simulink model "printer"  (R2017b)
settings: Solver=ode45  StartTime=0.0  StopTime=20  RelTol=1e-3  EnableMultiTasking=on
PreLoadFcn:
  | CONSTANTS
  | DEFAULT
  | System
  | Control
InitFcn:
  | CONSTANTS
  | DEFAULT
  | System
  | Control
values from neighbouring files (symbols this model uses):
  Amp0d = [C*L*R1 C*R1*R2]    [System.m]    (also in System_submitted.m = [Amp0d1 Amp0d0])
  Amp0n = [C*R1*R2-L]    [System.m]    (also in System_submitted.m = Amp0n0)
  Amp1d = Amp0d    [System.m]    (also in SystemHeadless.m; System_submitted.m)
  Amp1n = Amp0n    [System.m]    (also in SystemHeadless.m; System_submitted.m)
  AmpSat0 = MotorParam(NomV)    [System.m]    (also in SystemHeadless.m = q0(NomV); System_submitted.m = q0(NomV))
  AmpSat1 = Big    [System.m]    (also in SystemHeadless.m = AmpSat0; System_submitted.m = AmpSat0)
  BackEMF0 = 1/K_B    [System.m]    (also in SystemHeadless.m = 1 / q0(SpdK); System_submitted.m = 1 / q0(SpdK))
  BackEMF1 = 1/K_B1    [System.m]    (also in SystemHeadless.m = 1 / q1(SpdK); System_submitted.m = 1 / q1(SpdK))
  DegPerRad = 180/pi    (= 57.2957795131)    [CONSTANTS.m]
  Elec0d = [L_a R_a]    [System.m]    (also in SystemHeadless.m = [Elec0d1, Elec0d0]; System_submitted.m = [Elec0d1, Elec0d0])
  Elec0n = [1]    [System.m]    (also in SystemHeadless.m = 1; System_submitted.m = 1)
  Elec1d = [L_a R_a]    [System.m]    (also in SystemHeadless.m = [Elec1d1, Elec1d0]; System_submitted.m = [Elec1d1, Elec1d0])
  Elec1n = [1]    [System.m]    (also in SystemHeadless.m = 1; System_submitted.m = 1)
  JntSat1 = JntLim * RadPerDeg    [System.m]    (also in SystemHeadless.m = joint_limit; System_submitted.m = joint_limit)
  Mech0d = [J_system F_kf SpringK]    [System.m]    (also in SystemHeadless.m = [J_0, B_0, K_0]; System_submitted.m = [J_0, B_0, K_0])
  Mech0n = [1 0]    [System.m]    (also in SystemHeadless.m = [1, 0]; System_submitted.m = [1, 0])
  Mech1d = [J_rotor F_kf 0]    [System.m]    (also in SystemHeadless.m = [J_1, B_1, K_1]; System_submitted.m = [J_1, B_1, K_1])
  Mech1n = [1 0]    [System.m]    (also in SystemHeadless.m = [1, 0]; System_submitted.m = [1, 0])
  NomI0 = MotorParam(NomCurr)    [System.m]    (also in System_submitted.m = q0(NomCurr))
  NomI1 = MotorParam(NomCurr)    [System.m]    (also in System_submitted.m = q1(NomCurr))
  Sens0 = SensV / (SensAng * RadPerDeg)    [System.m]    (also in SystemHeadless.m; System_submitted.m)
  Sens1 = SensV / (SensAng * RadPerDeg)    [System.m]    (also in SystemHeadless.m; System_submitted.m)
  SensSat0 = SensV    [System.m]    (also in SystemHeadless.m; System_submitted.m)
  SensSat1 = SensV    [System.m]    (also in SystemHeadless.m; System_submitted.m)
  StallI0 = MotorParam(StallCurr)    [System.m]    (also in System_submitted.m = q0(StallCurr))
  StallI1 = MotorParam(StallCurr)    [System.m]    (also in System_submitted.m = q1(StallCurr))
  StFric0 = F_sf    [System.m]    (also in SystemHeadless.m = mu_SF * inner_fg; System_submitted.m = mu_SF * inner_fg)
  TConst0 = K_T    [System.m]    (also in SystemHeadless.m = q0(TorqueK); System_submitted.m = q0(TorqueK))
  TConst1 = K_T1    [System.m]    (also in SystemHeadless.m = q1(TorqueK); System_submitted.m = q1(TorqueK))
undefined symbols (not defined in the file or in its folder): FB0, FB1, Height, magnitude, PID0, PID1
libraries: simulink x22, vrlib x1
settings Model: Creator=Leos  LastModifiedBy=Moochster
settings DataIOCC: SaveFormat=Array
settings OptimizationCC: ExpressionDepthLimit=2147483647  LifeSpan=inf
settings DebuggingCC: UnderspecifiedInitializationDetection=Classic  MergeDetectMultiDrivingBlocksExec=none  SolverPrmCheckMsg=warning  FcnCallInpInsideContextMsg=warning  StateNameClashWarn=warning  SFUnexpectedBacktrackingDiag=warning  SFNoUnconditionalDefaultTransitionDiag=warning  SFExecutionAtInitializationDiag=none
settings HardwareCC: ProdBitPerPointer=32  ProdBitPerSizeT=32  ProdBitPerPtrDiffT=32  ProdLargestAtomicFloat=None  ProdIntDivRoundTo=Undefined  ProdEndianess=Unspecified  ProdWordSize=32  ProdHWDeviceType=32-bit Generic
settings ModelReferenceCC: PropagateSignalLabelsOutOfModel=off
settings CodeAppCC: StateflowObjectComments=on
settings GRTTargetCC: TargetLangStandard=C89/C90 (ANSI)  GeneratePreprocessorConditionals=Disable all  CombineOutputUpdateFcns=off  GRTInterface=on
settings ConfigComp: CovMetricSettings=dw  CovHtmlReporting=on  CovSaveCumulativeToWorkspaceVar=on  CovSaveSingleToWorkspaceVar=on  CovExternalEMLEnable=off  CovSFcnEnable=off

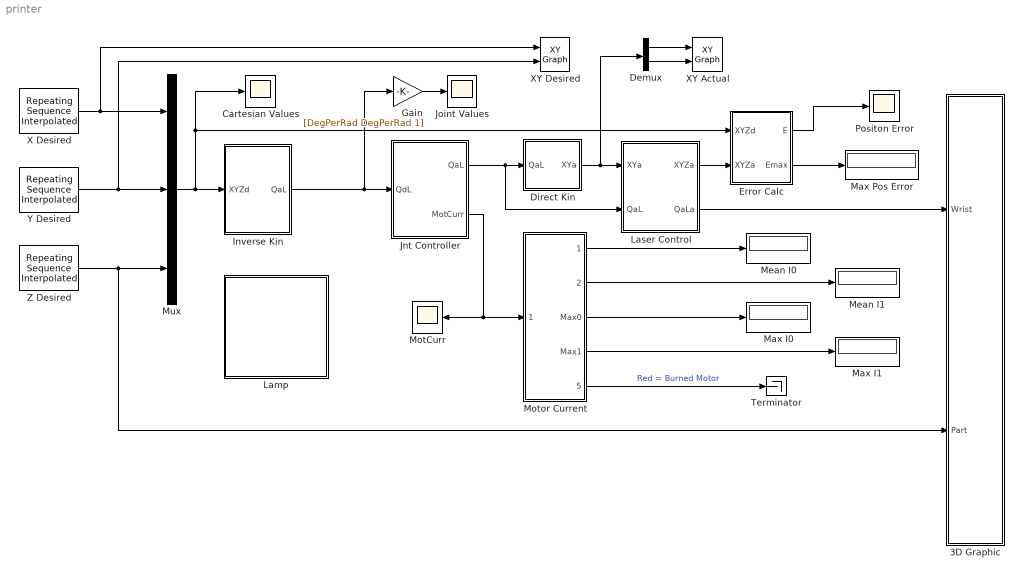
== system printer ==
  3D Graphic : Subsystem
  Cartesian Values : Scope
  Demux : Demux  Outputs=2
  Direct Kin : Subsystem
  Error Calc : Subsystem
  Gain : Gain  Gain=[DegPerRad DegPerRad 1]
  Inverse Kin : Subsystem
  Jnt Controller : Subsystem
  Joint Values : Scope
  Lamp : Subsystem  DialogController=hmiCreateDDGDialog  IsWebBlock=on  mask(MWDashboardBlock){webBlockId=7fcfd6b5-b98b-441a-9880-35fe4990fbef, webBlockType=lamp, ShowInLibBrowser=on, ShowInitialText=on, HMISrcModelName=printer}
      mask prompts: webBlockType "WebBlock Type"; HMISrcModelName "Source Model"
      mask help: SimulinkHMI:dialogs:LampDialogDesc
      mask Help: helpview([docroot '/mapfiles/simulink.map'], 'hmi_lamp')
      mask Display:
      | if strcmp(get_param(bdroot(gcb),'BlockDiagramType'), 'library')
      |     image([(matlabroot) '/toolbox/simulink/hmi/icons/Lamp.png']);
      | end
  Laser Control : Subsystem
  Max I0 : Display
  Max I1 : Display
  Max Pos Error : Display
  Mean I0 : Display
  Mean I1 : Display
  MotCurr : Scope
  Motor Current : Subsystem
  Mux : Mux  Inputs=3
  Positon Error : Scope
  Terminator : Terminator
  X Desired : simulink/Sources/Repeating Sequence Interpolated  OutValues=Xd  TimeValues=Time  LookUpMeth=Interpolation-Use End Values  tsamp=SampleTime  OutMin=[]  OutMax=[]  OutDataTypeStr=double  OutputDataTypeScalingMode=double  OutDataType=fixdt(0,8)  OutScaling=2^-10
  "XY Actual " : simulink/Sinks/XY Graph  xmin=-110  xmax=110  ymin=-110  ymax=110  st=-1
  XY Desired : simulink/Sinks/XY Graph  xmin=-110  xmax=110  ymin=-110  ymax=110  st=-1
  Y Desired : simulink/Sources/Repeating Sequence Interpolated  OutValues=Yd  TimeValues=Time  LookUpMeth=Interpolation-Use End Values  tsamp=SampleTime  OutMin=[]  OutMax=[]  OutDataTypeStr=double  OutputDataTypeScalingMode=double  OutDataType=fixdt(0,8)  OutScaling=2^-10
  Z Desired : simulink/Sources/Repeating Sequence Interpolated  OutValues=Zd  TimeValues=Time  LookUpMeth=Interpolation-Use End Values  tsamp=SampleTime  OutMin=[]  OutMax=[]  OutDataTypeStr=double  OutputDataTypeScalingMode=double  OutDataType=fixdt(0,8)  OutScaling=2^-10
  wires:
  Inverse Kin/1(QaL) -> Gain/1, Jnt Controller/1(QdL)
  Y Desired/1 -> XY Desired/2, Mux/2
  X Desired/1 -> Mux/1, XY Desired/1
  Demux/2 -> "XY Actual "/2
  Direct Kin/1(XYa) -> Demux/1, Laser Control/1(XYa)
  Demux/1 -> "XY Actual "/1
  Z Desired/1 -> 3D Graphic/2(Part), Mux/3
  Laser Control/2(QaLa) -> 3D Graphic/1(Wrist)
  Mux/1 -> Error Calc/1(XYZd), Cartesian Values/1, Inverse Kin/1(XYZd)
  Laser Control/1(XYZa) -> Error Calc/2(XYZa)
  Error Calc/2(Emax) -> Max Pos Error/1
  Error Calc/1(E) -> Positon Error/1
  Jnt Controller/2(MotCurr) -> MotCurr/1, Motor Current/1(MotCurr)
  Motor Current/1(Mean0) -> Mean I0/1
  Motor Current/4(Max1) -> Max I1/1
  Gain/1 -> Joint Values/1
  Motor Current/3(Max0) -> Max I0/1
  Motor Current/2(Mean1) -> Mean I1/1
  Motor Current/5(Burned) -> Terminator/1  "Red = Burned Motor"
  Jnt Controller/1(QaL) -> Direct Kin/1(QaL), Laser Control/2(QaL)

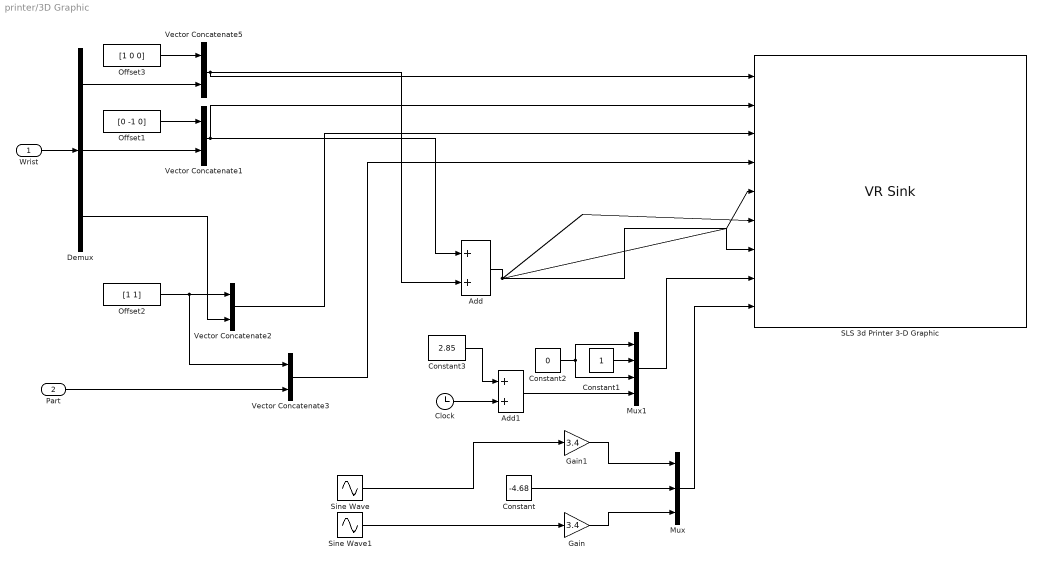
== system printer/3D Graphic ==
  Wrist : Inport
  Part : Inport  Port=2
  Add : Sum
  Add1 : Sum
  Clock : Clock
  Constant : Constant  Value=-4.68
  Constant1 : Constant
  Constant2 : Constant  Value=0
  Constant3 : Constant  Value=2.85
  Demux : Demux  Outputs=3
  Gain : Gain  Gain=3.4
  Gain1 : Gain  Gain=3.4
  Mux : Mux  Inputs=3
  Mux1 : Mux
  Offset1 : Constant  Value=[0 -1 0]
  Offset2 : Constant  Value=[1 1]
  Offset3 : Constant  Value=[1 0 0]
  SLS 3d Printer 3-D Graphic : vrlib/VR Sink  InstantiateOnLoad=on  SampleTime=0.01  ViewEnable=on  RemoteChange=off  RemoteView=off  FieldsWritten=q1.rotation.4.1.1.double#q2.rotation.4.1.1.double#LaserBeam.scale.3.1.1.double#Part.scale.3.1.1.double#HandL.rotation.4.1.1.double#ArmL.rotation.4.1.1.double#SleeveL.rotation.4.1.1.double#Fish.rotation.4.1.1.double#Fish.translation.3.1.1.double  WorldFileName=3dPrinter.WRL  AutoView=on  VideoDimensions=[]  AllowVariableSize=off
      settings: SourceProductBaseCode=VR
  Sine Wave : Sin  SampleTime=0
  Sine Wave1 : Sin  Phase=1.571  SampleTime=0
  Vector Concatenate{1..3,5} (4 alike) : Concatenate
  wires:
  Demux/1 -> Vector Concatenate5/2
  Demux/2 -> Vector Concatenate1/2
  Offset3/1 -> Vector Concatenate5/1
  Offset1/1 -> Vector Concatenate1/1
  Wrist/1 -> Demux/1
  Offset2/1 -> Vector Concatenate3/1, Vector Concatenate2/1
  Part/1 -> Vector Concatenate3/2
  Demux/3 -> Vector Concatenate2/2
  Vector Concatenate5/1 -> Add/2, SLS 3d Printer 3-D Graphic/1
  Vector Concatenate1/1 -> Add/1, SLS 3d Printer 3-D Graphic/2
  Vector Concatenate2/1 -> SLS 3d Printer 3-D Graphic/3
  Vector Concatenate3/1 -> SLS 3d Printer 3-D Graphic/4
  Add/1 -> SLS 3d Printer 3-D Graphic/5, SLS 3d Printer 3-D Graphic/6, SLS 3d Printer 3-D Graphic/7
  Constant/1 -> Mux/2
  Sine Wave/1 -> Gain1/1
  Sine Wave1/1 -> Gain/1
  Mux/1 -> SLS 3d Printer 3-D Graphic/9
  Constant1/1 -> Mux1/2
  Constant2/1 -> Mux1/3, Mux1/1
  Mux1/1 -> SLS 3d Printer 3-D Graphic/8
  Add1/1 -> Mux1/4
  Constant3/1 -> Add1/1
  Gain/1 -> Mux/3
  Gain1/1 -> Mux/1
  Clock/1 -> Add1/2

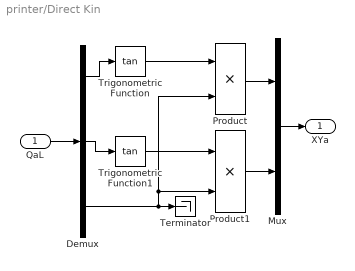
== system printer/Direct Kin ==
  QaL : Inport
  Demux : Demux  Outputs=3
  Mux : Mux  Inputs=2
  Product : Product
  Product1 : Product
  Terminator : Terminator
  Trigonometric Function : Trigonometry  Operator=tan
  Trigonometric Function1 : Trigonometry  Operator=tan
  XYa : Outport
  wires:
  QaL/1 -> Demux/1
  Mux/1 -> XYa/1
  Demux/1 -> Trigonometric Function/1
  Demux/2 -> Trigonometric Function1/1
  Demux/3 -> Terminator/1, Product/2, Product1/2
  Trigonometric Function/1 -> Product/1
  Product/1 -> Mux/1
  Product1/1 -> Mux/2
  Trigonometric Function1/1 -> Product1/1

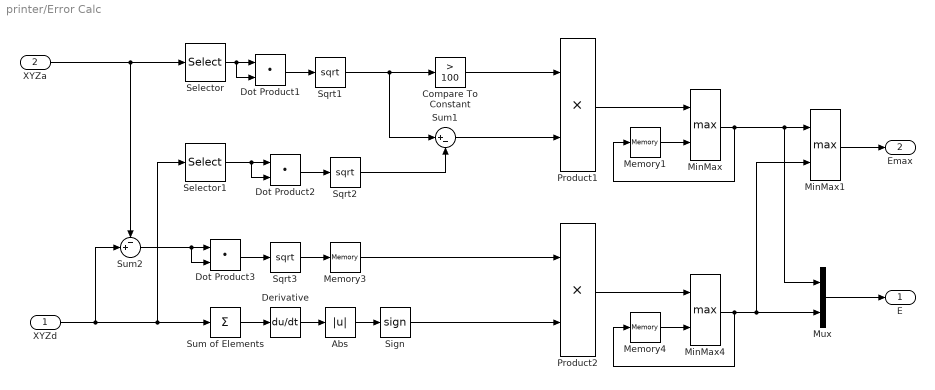
== system printer/Error Calc ==
  XYZd : Inport
  XYZa : Inport  Port=2
  Abs : Abs
  Compare To Constant : simulink/Logic and Bit Operations/Compare To Constant  relop=>  const=100  OutDataTypeStr=boolean
  Derivative : Derivative
  Dot Product1 : DotProduct  InputSameDT=on  OutDataTypeStr=Inherit: Inherit via internal rule
  Dot Product2 : DotProduct  InputSameDT=on  OutDataTypeStr=Inherit: Inherit via internal rule
  Dot Product3 : DotProduct  InputSameDT=on  OutDataTypeStr=Inherit: Inherit via internal rule
  Memory1 : Memory
  Memory3 : Memory
  Memory4 : Memory
  MinMax : MinMax  Function=max  Inputs=2
  MinMax1 : MinMax  Function=max  Inputs=2
  MinMax4 : MinMax  Function=max  Inputs=2
  Mux : Mux  Inputs=2
  Product1 : Product
  Product2 : Product
  Selector : Selector  InputPortWidth=3  IndexOptions=Index vector (dialog)  Indices=[1 2]  OutputSizes=1
  Selector1 : Selector  InputPortWidth=3  IndexOptions=Index vector (dialog)  Indices=[1 2]  OutputSizes=1
  Sign : Signum
  Sqrt1 : Sqrt  SaturateOnIntegerOverflow=on
  Sqrt2 : Sqrt  SaturateOnIntegerOverflow=on
  Sqrt3 : Sqrt  SaturateOnIntegerOverflow=on
  Sum of Elements : Sum  Inputs=+
  Sum1 : Sum  Inputs=|+-
  Sum2 : Sum  Inputs=-+|
  E : Outport
  Emax : Outport  Port=2
  wires:
  XYZd/1 -> Sum2/2, Selector1/1, Sum of Elements/1
  Derivative/1 -> Abs/1
  Abs/1 -> Sign/1
  Sum of Elements/1 -> Derivative/1
  Selector/1 -> Dot Product1/2, Dot Product1/1
  Dot Product1/1 -> Sqrt1/1
  XYZa/1 -> Sum2/1, Selector/1
  Sign/1 -> Product2/2
  Sqrt1/1 -> Sum1/1, Compare To Constant/1
  Product1/1 -> MinMax/1
  Compare To Constant/1 -> Product1/1
  Sum1/1 -> Product1/2
  Memory1/1 -> MinMax/2
  MinMax/1 -> Mux/1, MinMax1/1, Memory1/1
  Memory4/1 -> MinMax4/2
  Product2/1 -> MinMax4/1
  MinMax4/1 -> MinMax1/2, Mux/2, Memory4/1
  MinMax1/1 -> Emax/1
  Mux/1 -> E/1
  Memory3/1 -> Product2/1
  Selector1/1 -> Dot Product2/2, Dot Product2/1
  Dot Product2/1 -> Sqrt2/1
  Sqrt2/1 -> Sum1/2
  Sum2/1 -> Dot Product3/2, Dot Product3/1
  Dot Product3/1 -> Sqrt3/1
  Sqrt3/1 -> Memory3/1

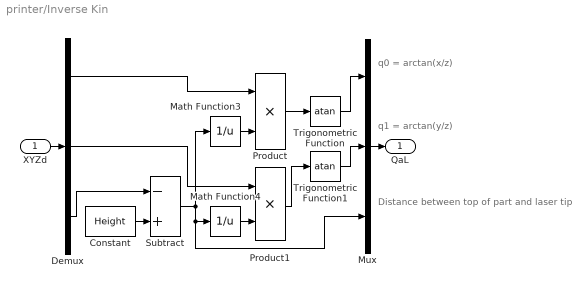
== system printer/Inverse Kin ==
  note: Distance between top of part and laser tip
  note: q0 = arctan(x/z)
  note: q1 = arctan(y/z)
  XYZd : Inport
  Constant : Constant  Value=Height
  Demux : Demux  Outputs=3
  Math Function3 : Math  Operator=reciprocal  SaturateOnIntegerOverflow=on
  Math Function4 : Math  Operator=reciprocal  SaturateOnIntegerOverflow=on
  Mux : Mux  Inputs=3
  Product : Product
  Product1 : Product
  Subtract : Sum  Inputs=-+
  Trigonometric Function : Trigonometry  Operator=atan
  Trigonometric Function1 : Trigonometry  Operator=atan
  QaL : Outport
  wires:
  XYZd/1 -> Demux/1
  Mux/1 -> QaL/1
  Demux/1 -> Product/1
  Demux/2 -> Product1/1
  Demux/3 -> Subtract/1
  Trigonometric Function/1 -> Mux/1
  Trigonometric Function1/1 -> Mux/2
  Constant/1 -> Subtract/2
  Product/1 -> Trigonometric Function/1
  Product1/1 -> Trigonometric Function1/1
  Math Function3/1 -> Product/2
  Math Function4/1 -> Product1/2
  Subtract/1 -> Math Function3/1, Math Function4/1, Mux/3

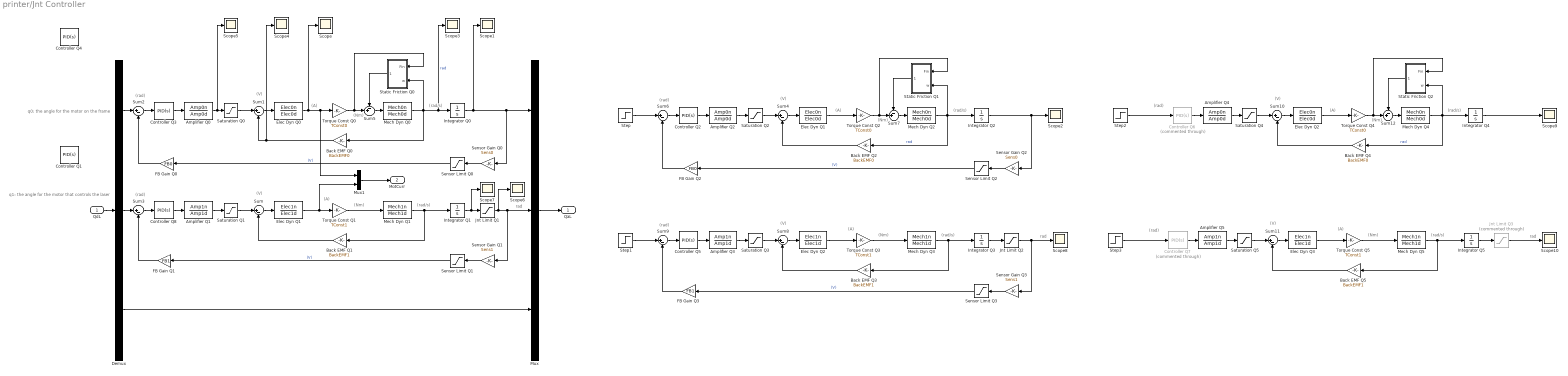
== system printer/Jnt Controller ==
  note: rad
  note: (rad/s)
  note: (V)
  note: (rad)
  note: (A)
  note: (Nm)
  note: (rad/s)
  note: (V)
  note: (rad)
  note: (A)
  note: (Nm)
  note: q0: the angle for the motor on the frame
  note: q1: the angle for the motor that controls the laser
  note: (Nm)
  note: (rad/s)
  note: (V)
  note: (rad)
  note: (A)
  note: (A)
  note: (rad)
  note: (V)
  note: (rad/s)
  note: rad
  note: (Nm)
  note: (A)
  note: (Nm)
  note: (rad)
  note: (rad/s)
  note: (V)
  note: (rad)
  note: (Nm)
  note: (A)
  note: rad
  note: (rad/s)
  note: (V)
  QdL : Inport
  Amplifier Q0 : TransferFcn  Numerator=Amp0n  Denominator=Amp0d
  Amplifier Q1 : TransferFcn  Numerator=Amp1n  Denominator=Amp1d
  Amplifier Q2 : TransferFcn  Numerator=Amp0n  Denominator=Amp0d
  Amplifier Q3 : TransferFcn  Numerator=Amp1n  Denominator=Amp1d
  Amplifier Q4 : TransferFcn  Numerator=Amp0n  Denominator=Amp0d
  Amplifier Q5 : TransferFcn  Numerator=Amp1n  Denominator=Amp1d
  Back EMF Q0 : Gain  Gain=BackEMF0
  Back EMF Q1 : Gain  Gain=BackEMF1
  Back EMF Q2 : Gain  Gain=BackEMF0
  Back EMF Q3 : Gain  Gain=BackEMF1
  Back EMF Q4 : Gain  Gain=BackEMF0
  Back EMF Q5 : Gain  Gain=BackEMF1
  Controller Q1 : simulink/Continuous/PID Controller  Controller=PID  TimeDomain=Continuous-time  SampleTime=-1  IntegratorMethod=Forward Euler  FilterMethod=Forward Euler  Form=Parallel  UseFilter=on  ControllerParametersSource=internal  P=0.325398300430713  I=1.13628459398882  D=0.0191166653473395  N=7531.30108660087  InitialConditionSource=internal  InitialConditionForIntegrator=0  InitialConditionForFilter=0  ExternalReset=none  LimitOutput=off  UpperSaturationLimit=inf  LowerSaturationLimit=-inf  LinearizeAsGain=on  AntiWindupMode=none  Kb=1  TrackingMode=off  Kt=1  PParamMin=[]  PParamMax=[]  IParamMin=[]  IParamMax=[]  DParamMin=[]  DParamMax=[]  NParamMin=[]  NParamMax=[]  KbParamMin=[]  KbParamMax=[]  KtParamMin=[]  KtParamMax=[]  POutMin=[]  POutMax=[]  IOutMin=[]  IOutMax=[]  DOutMin=[]  DOutMax=[]  NOutMin=[]  NOutMax=[]  KbOutMin=[]  KbOutMax=[]  KtOutMin=[]  KtOutMax=[]  IntegratorOutMin=[]  IntegratorOutMax=[]  FilterOutMin=[]  FilterOutMax=[]  SumOutMin=[]  SumOutMax=[]  SumI1OutMin=[]  SumI1OutMax=[]  SumI2OutMin=[]  SumI2OutMax=[]  SumI3OutMin=[]  SumI3OutMax=[]  SumDOutMin=[]  SumDOutMax=[]  SaturationOutMin=[]  SaturationOutMax=[]  IntegratorContinuousStateAttributes=''  IntegratorStateMustResolveToSignalObject=off  IntegratorRTWStateStorageClass=Auto  FilterContinuousStateAttributes=''  FilterStateMustResolveToSignalObject=off  FilterRTWStateStorageClass=Auto  DifferentiatorICPrevScaledInput=0  DifferentiatorOutMin=[]  DifferentiatorOutMax=[]  InitialConditionSetting=State (most efficient)  FilterDiffOutCoefMin=[]  FilterDiffOutCoefMax=[]  SumDenOutMin=[]  SumDenOutMax=[]  SumNumOutMin=[]  SumNumOutMax=[]  ReciprocalOutMin=[]  ReciprocalOutMax=[]  DivideOutMin=[]  DivideOutMax=[]  TunerSelectOption=Transfer Function Based (PID Tuner App)
  Controller Q2 : simulink/Continuous/PID Controller  Controller=PID  TimeDomain=Continuous-time  SampleTime=-1  IntegratorMethod=Forward Euler  FilterMethod=Forward Euler  Form=Parallel  UseFilter=on  ControllerParametersSource=internal  P=PID0(1)  I=PID0(2)  D=PID0(3)  N=100  InitialConditionSource=internal  InitialConditionForIntegrator=0  InitialConditionForFilter=0  ExternalReset=none  LimitOutput=off  UpperSaturationLimit=inf  LowerSaturationLimit=-inf  LinearizeAsGain=on  AntiWindupMode=none  Kb=1  TrackingMode=off  Kt=1  PParamMin=[]  PParamMax=[]  IParamMin=[]  IParamMax=[]  DParamMin=[]  DParamMax=[]  NParamMin=[]  NParamMax=[]  KbParamMin=[]  KbParamMax=[]  KtParamMin=[]  KtParamMax=[]  POutMin=[]  POutMax=[]  IOutMin=[]  IOutMax=[]  DOutMin=[]  DOutMax=[]  NOutMin=[]  NOutMax=[]  KbOutMin=[]  KbOutMax=[]  KtOutMin=[]  KtOutMax=[]  IntegratorOutMin=[]  IntegratorOutMax=[]  FilterOutMin=[]  FilterOutMax=[]  SumOutMin=[]  SumOutMax=[]  SumI1OutMin=[]  SumI1OutMax=[]  SumI2OutMin=[]  SumI2OutMax=[]  SumI3OutMin=[]  SumI3OutMax=[]  SumDOutMin=[]  SumDOutMax=[]  SaturationOutMin=[]  SaturationOutMax=[]  IntegratorContinuousStateAttributes=''  IntegratorStateMustResolveToSignalObject=off  IntegratorRTWStateStorageClass=Auto  FilterContinuousStateAttributes=''  FilterStateMustResolveToSignalObject=off  FilterRTWStateStorageClass=Auto  DifferentiatorICPrevScaledInput=0  DifferentiatorOutMin=[]  DifferentiatorOutMax=[]  InitialConditionSetting=State (most efficient)  FilterDiffOutCoefMin=[]  FilterDiffOutCoefMax=[]  SumDenOutMin=[]  SumDenOutMax=[]  SumNumOutMin=[]  SumNumOutMax=[]  ReciprocalOutMin=[]  ReciprocalOutMax=[]  DivideOutMin=[]  DivideOutMax=[]  TunerSelectOption=Transfer Function Based (PID Tuner App)
  Controller Q3 : simulink/Continuous/PID Controller  Controller=PID  TimeDomain=Continuous-time  SampleTime=-1  IntegratorMethod=Forward Euler  FilterMethod=Forward Euler  Form=Parallel  UseFilter=on  ControllerParametersSource=internal  P=PID0(1)  I=PID0(2)  D=PID0(3)  N=100  InitialConditionSource=internal  InitialConditionForIntegrator=0  InitialConditionForFilter=0  ExternalReset=none  LimitOutput=off  UpperSaturationLimit=inf  LowerSaturationLimit=-inf  LinearizeAsGain=on  AntiWindupMode=none  Kb=1  TrackingMode=off  Kt=1  PParamMin=[]  PParamMax=[]  IParamMin=[]  IParamMax=[]  DParamMin=[]  DParamMax=[]  NParamMin=[]  NParamMax=[]  KbParamMin=[]  KbParamMax=[]  KtParamMin=[]  KtParamMax=[]  POutMin=[]  POutMax=[]  IOutMin=[]  IOutMax=[]  DOutMin=[]  DOutMax=[]  NOutMin=[]  NOutMax=[]  KbOutMin=[]  KbOutMax=[]  KtOutMin=[]  KtOutMax=[]  IntegratorOutMin=[]  IntegratorOutMax=[]  FilterOutMin=[]  FilterOutMax=[]  SumOutMin=[]  SumOutMax=[]  SumI1OutMin=[]  SumI1OutMax=[]  SumI2OutMin=[]  SumI2OutMax=[]  SumI3OutMin=[]  SumI3OutMax=[]  SumDOutMin=[]  SumDOutMax=[]  SaturationOutMin=[]  SaturationOutMax=[]  IntegratorContinuousStateAttributes=''  IntegratorStateMustResolveToSignalObject=off  IntegratorRTWStateStorageClass=Auto  FilterContinuousStateAttributes=''  FilterStateMustResolveToSignalObject=off  FilterRTWStateStorageClass=Auto  DifferentiatorICPrevScaledInput=0  DifferentiatorOutMin=[]  DifferentiatorOutMax=[]  InitialConditionSetting=State (most efficient)  FilterDiffOutCoefMin=[]  FilterDiffOutCoefMax=[]  SumDenOutMin=[]  SumDenOutMax=[]  SumNumOutMin=[]  SumNumOutMax=[]  ReciprocalOutMin=[]  ReciprocalOutMax=[]  DivideOutMin=[]  DivideOutMax=[]  TunerSelectOption=Transfer Function Based (PID Tuner App)
  Controller Q4 : simulink/Continuous/PID Controller  Controller=PID  TimeDomain=Continuous-time  SampleTime=-1  IntegratorMethod=Forward Euler  FilterMethod=Forward Euler  Form=Parallel  UseFilter=on  ControllerParametersSource=internal  P=3.19495744260721  I=12.8018971006006  D=0.15685788274795  N=317.014850980507  InitialConditionSource=internal  InitialConditionForIntegrator=0  InitialConditionForFilter=0  ExternalReset=none  LimitOutput=off  UpperSaturationLimit=inf  LowerSaturationLimit=-inf  LinearizeAsGain=on  AntiWindupMode=none  Kb=1  TrackingMode=off  Kt=1  PParamMin=[]  PParamMax=[]  IParamMin=[]  IParamMax=[]  DParamMin=[]  DParamMax=[]  NParamMin=[]  NParamMax=[]  KbParamMin=[]  KbParamMax=[]  KtParamMin=[]  KtParamMax=[]  POutMin=[]  POutMax=[]  IOutMin=[]  IOutMax=[]  DOutMin=[]  DOutMax=[]  NOutMin=[]  NOutMax=[]  KbOutMin=[]  KbOutMax=[]  KtOutMin=[]  KtOutMax=[]  IntegratorOutMin=[]  IntegratorOutMax=[]  FilterOutMin=[]  FilterOutMax=[]  SumOutMin=[]  SumOutMax=[]  SumI1OutMin=[]  SumI1OutMax=[]  SumI2OutMin=[]  SumI2OutMax=[]  SumI3OutMin=[]  SumI3OutMax=[]  SumDOutMin=[]  SumDOutMax=[]  SaturationOutMin=[]  SaturationOutMax=[]  IntegratorContinuousStateAttributes=''  IntegratorStateMustResolveToSignalObject=off  IntegratorRTWStateStorageClass=Auto  FilterContinuousStateAttributes=''  FilterStateMustResolveToSignalObject=off  FilterRTWStateStorageClass=Auto  DifferentiatorICPrevScaledInput=0  DifferentiatorOutMin=[]  DifferentiatorOutMax=[]  InitialConditionSetting=State (most efficient)  FilterDiffOutCoefMin=[]  FilterDiffOutCoefMax=[]  SumDenOutMin=[]  SumDenOutMax=[]  SumNumOutMin=[]  SumNumOutMax=[]  ReciprocalOutMin=[]  ReciprocalOutMax=[]  DivideOutMin=[]  DivideOutMax=[]  TunerSelectOption=Transfer Function Based (PID Tuner App)
  Controller Q5 : simulink/Continuous/PID Controller  Controller=PID  TimeDomain=Continuous-time  SampleTime=-1  IntegratorMethod=Forward Euler  FilterMethod=Forward Euler  Form=Parallel  UseFilter=on  ControllerParametersSource=internal  P=PID1(1)  I=PID1(2)  D=PID1(3)  N=100  InitialConditionSource=internal  InitialConditionForIntegrator=0  InitialConditionForFilter=0  ExternalReset=none  LimitOutput=off  UpperSaturationLimit=inf  LowerSaturationLimit=-inf  LinearizeAsGain=on  AntiWindupMode=none  Kb=1  TrackingMode=off  Kt=1  PParamMin=[]  PParamMax=[]  IParamMin=[]  IParamMax=[]  DParamMin=[]  DParamMax=[]  NParamMin=[]  NParamMax=[]  KbParamMin=[]  KbParamMax=[]  KtParamMin=[]  KtParamMax=[]  POutMin=[]  POutMax=[]  IOutMin=[]  IOutMax=[]  DOutMin=[]  DOutMax=[]  NOutMin=[]  NOutMax=[]  KbOutMin=[]  KbOutMax=[]  KtOutMin=[]  KtOutMax=[]  IntegratorOutMin=[]  IntegratorOutMax=[]  FilterOutMin=[]  FilterOutMax=[]  SumOutMin=[]  SumOutMax=[]  SumI1OutMin=[]  SumI1OutMax=[]  SumI2OutMin=[]  SumI2OutMax=[]  SumI3OutMin=[]  SumI3OutMax=[]  SumDOutMin=[]  SumDOutMax=[]  SaturationOutMin=[]  SaturationOutMax=[]  IntegratorContinuousStateAttributes=''  IntegratorStateMustResolveToSignalObject=off  IntegratorRTWStateStorageClass=Auto  FilterContinuousStateAttributes=''  FilterStateMustResolveToSignalObject=off  FilterRTWStateStorageClass=Auto  DifferentiatorICPrevScaledInput=0  DifferentiatorOutMin=[]  DifferentiatorOutMax=[]  InitialConditionSetting=State (most efficient)  FilterDiffOutCoefMin=[]  FilterDiffOutCoefMax=[]  SumDenOutMin=[]  SumDenOutMax=[]  SumNumOutMin=[]  SumNumOutMax=[]  ReciprocalOutMin=[]  ReciprocalOutMax=[]  DivideOutMin=[]  DivideOutMax=[]  TunerSelectOption=Transfer Function Based (PID Tuner App)
  Controller Q6 : simulink/Continuous/PID Controller  Commented=through  Controller=PID  TimeDomain=Continuous-time  SampleTime=-1  IntegratorMethod=Forward Euler  FilterMethod=Forward Euler  Form=Parallel  UseFilter=on  ControllerParametersSource=internal  P=1.5024184383397  I=5.78181210407204  D=0.097054291994374  N=2502.8130936281  InitialConditionSource=internal  InitialConditionForIntegrator=0  InitialConditionForFilter=0  ExternalReset=none  LimitOutput=off  UpperSaturationLimit=inf  LowerSaturationLimit=-inf  LinearizeAsGain=on  AntiWindupMode=none  Kb=1  TrackingMode=off  Kt=1  PParamMin=[]  PParamMax=[]  IParamMin=[]  IParamMax=[]  DParamMin=[]  DParamMax=[]  NParamMin=[]  NParamMax=[]  KbParamMin=[]  KbParamMax=[]  KtParamMin=[]  KtParamMax=[]  POutMin=[]  POutMax=[]  IOutMin=[]  IOutMax=[]  DOutMin=[]  DOutMax=[]  NOutMin=[]  NOutMax=[]  KbOutMin=[]  KbOutMax=[]  KtOutMin=[]  KtOutMax=[]  IntegratorOutMin=[]  IntegratorOutMax=[]  FilterOutMin=[]  FilterOutMax=[]  SumOutMin=[]  SumOutMax=[]  SumI1OutMin=[]  SumI1OutMax=[]  SumI2OutMin=[]  SumI2OutMax=[]  SumI3OutMin=[]  SumI3OutMax=[]  SumDOutMin=[]  SumDOutMax=[]  SaturationOutMin=[]  SaturationOutMax=[]  IntegratorContinuousStateAttributes=''  IntegratorStateMustResolveToSignalObject=off  IntegratorRTWStateStorageClass=Auto  FilterContinuousStateAttributes=''  FilterStateMustResolveToSignalObject=off  FilterRTWStateStorageClass=Auto  DifferentiatorICPrevScaledInput=0  DifferentiatorOutMin=[]  DifferentiatorOutMax=[]  InitialConditionSetting=State (most efficient)  FilterDiffOutCoefMin=[]  FilterDiffOutCoefMax=[]  SumDenOutMin=[]  SumDenOutMax=[]  SumNumOutMin=[]  SumNumOutMax=[]  ReciprocalOutMin=[]  ReciprocalOutMax=[]  DivideOutMin=[]  DivideOutMax=[]  TunerSelectOption=Transfer Function Based (PID Tuner App)
  Controller Q7 : simulink/Continuous/PID Controller  Commented=through  Controller=PID  TimeDomain=Continuous-time  SampleTime=-1  IntegratorMethod=Forward Euler  FilterMethod=Forward Euler  Form=Parallel  UseFilter=on  ControllerParametersSource=internal  P=0.183181513146469  I=0.345187772411702  D=0.0108464673507805  N=4538.05766534358  InitialConditionSource=internal  InitialConditionForIntegrator=0  InitialConditionForFilter=0  ExternalReset=none  LimitOutput=off  UpperSaturationLimit=inf  LowerSaturationLimit=-inf  LinearizeAsGain=on  AntiWindupMode=none  Kb=1  TrackingMode=off  Kt=1  PParamMin=[]  PParamMax=[]  IParamMin=[]  IParamMax=[]  DParamMin=[]  DParamMax=[]  NParamMin=[]  NParamMax=[]  KbParamMin=[]  KbParamMax=[]  KtParamMin=[]  KtParamMax=[]  POutMin=[]  POutMax=[]  IOutMin=[]  IOutMax=[]  DOutMin=[]  DOutMax=[]  NOutMin=[]  NOutMax=[]  KbOutMin=[]  KbOutMax=[]  KtOutMin=[]  KtOutMax=[]  IntegratorOutMin=[]  IntegratorOutMax=[]  FilterOutMin=[]  FilterOutMax=[]  SumOutMin=[]  SumOutMax=[]  SumI1OutMin=[]  SumI1OutMax=[]  SumI2OutMin=[]  SumI2OutMax=[]  SumI3OutMin=[]  SumI3OutMax=[]  SumDOutMin=[]  SumDOutMax=[]  SaturationOutMin=[]  SaturationOutMax=[]  IntegratorContinuousStateAttributes=''  IntegratorStateMustResolveToSignalObject=off  IntegratorRTWStateStorageClass=Auto  FilterContinuousStateAttributes=''  FilterStateMustResolveToSignalObject=off  FilterRTWStateStorageClass=Auto  DifferentiatorICPrevScaledInput=0  DifferentiatorOutMin=[]  DifferentiatorOutMax=[]  InitialConditionSetting=State (most efficient)  FilterDiffOutCoefMin=[]  FilterDiffOutCoefMax=[]  SumDenOutMin=[]  SumDenOutMax=[]  SumNumOutMin=[]  SumNumOutMax=[]  ReciprocalOutMin=[]  ReciprocalOutMax=[]  DivideOutMin=[]  DivideOutMax=[]  TunerSelectOption=Transfer Function Based (PID Tuner App)
  Controller Q8 : simulink/Continuous/PID Controller  Controller=PID  TimeDomain=Continuous-time  SampleTime=-1  IntegratorMethod=Forward Euler  FilterMethod=Forward Euler  Form=Parallel  UseFilter=on  ControllerParametersSource=internal  P=PID1(1)  I=PID1(2)  D=PID1(3)  N=100  InitialConditionSource=internal  InitialConditionForIntegrator=0  InitialConditionForFilter=0  ExternalReset=none  LimitOutput=off  UpperSaturationLimit=inf  LowerSaturationLimit=-inf  LinearizeAsGain=on  AntiWindupMode=none  Kb=1  TrackingMode=off  Kt=1  PParamMin=[]  PParamMax=[]  IParamMin=[]  IParamMax=[]  DParamMin=[]  DParamMax=[]  NParamMin=[]  NParamMax=[]  KbParamMin=[]  KbParamMax=[]  KtParamMin=[]  KtParamMax=[]  POutMin=[]  POutMax=[]  IOutMin=[]  IOutMax=[]  DOutMin=[]  DOutMax=[]  NOutMin=[]  NOutMax=[]  KbOutMin=[]  KbOutMax=[]  KtOutMin=[]  KtOutMax=[]  IntegratorOutMin=[]  IntegratorOutMax=[]  FilterOutMin=[]  FilterOutMax=[]  SumOutMin=[]  SumOutMax=[]  SumI1OutMin=[]  SumI1OutMax=[]  SumI2OutMin=[]  SumI2OutMax=[]  SumI3OutMin=[]  SumI3OutMax=[]  SumDOutMin=[]  SumDOutMax=[]  SaturationOutMin=[]  SaturationOutMax=[]  IntegratorContinuousStateAttributes=''  IntegratorStateMustResolveToSignalObject=off  IntegratorRTWStateStorageClass=Auto  FilterContinuousStateAttributes=''  FilterStateMustResolveToSignalObject=off  FilterRTWStateStorageClass=Auto  DifferentiatorICPrevScaledInput=0  DifferentiatorOutMin=[]  DifferentiatorOutMax=[]  InitialConditionSetting=State (most efficient)  FilterDiffOutCoefMin=[]  FilterDiffOutCoefMax=[]  SumDenOutMin=[]  SumDenOutMax=[]  SumNumOutMin=[]  SumNumOutMax=[]  ReciprocalOutMin=[]  ReciprocalOutMax=[]  DivideOutMin=[]  DivideOutMax=[]  TunerSelectOption=Transfer Function Based (PID Tuner App)
  Demux : Demux  Outputs=3
  Elec Dyn Q0 : TransferFcn  Numerator=Elec0n  Denominator=Elec0d
  Elec Dyn Q1 : TransferFcn  Numerator=Elec0n  Denominator=Elec0d
  Elec Dyn Q2 : TransferFcn  Numerator=Elec0n  Denominator=Elec0d
  Elec Dyn Q1 : TransferFcn  Numerator=Elec1n  Denominator=Elec1d
  Elec Dyn Q2 : TransferFcn  Numerator=Elec1n  Denominator=Elec1d
  Elec Dyn Q3 : TransferFcn  Numerator=Elec1n  Denominator=Elec1d
  FB Gain Q0 : Gain  Gain=FB0
  FB Gain Q1 : Gain  Gain=FB1
  FB Gain Q2 : Gain  Gain=FB0
  FB Gain Q3 : Gain  Gain=FB1
  Integrator Q{0..5} (6 alike) : Integrator
  Jnt Limit Q1 : Saturate  UpperLimit=JntSat1  LowerLimit=-JntSat1
  Jnt Limit Q2 : Saturate  UpperLimit=JntSat1  LowerLimit=-JntSat1
  Jnt Limit Q3 : Saturate  Commented=through  UpperLimit=JntSat1  LowerLimit=-JntSat1
  Mech Dyn Q0 : TransferFcn  Numerator=Mech0n  Denominator=Mech0d
  Mech Dyn Q1 : TransferFcn  Numerator=Mech1n  Denominator=Mech1d
  Mech Dyn Q2 : TransferFcn  Numerator=Mech0n  Denominator=Mech0d
  Mech Dyn Q3 : TransferFcn  Numerator=Mech1n  Denominator=Mech1d
  Mech Dyn Q4 : TransferFcn  Numerator=Mech0n  Denominator=Mech0d
  Mech Dyn Q5 : TransferFcn  Numerator=Mech1n  Denominator=Mech1d
  Mux : Mux  Inputs=3
  Mux1 : Mux  Inputs=2
  Saturation Q0 : Saturate  UpperLimit=AmpSat0  LowerLimit=-AmpSat0
  Saturation Q1 : Saturate  UpperLimit=AmpSat1  LowerLimit=-AmpSat1
  Saturation Q2 : Saturate  UpperLimit=AmpSat0  LowerLimit=-AmpSat0
  Saturation Q3 : Saturate  UpperLimit=AmpSat1  LowerLimit=-AmpSat1
  Saturation Q4 : Saturate  UpperLimit=AmpSat0  LowerLimit=-AmpSat0
  Saturation Q5 : Saturate  UpperLimit=AmpSat1  LowerLimit=-AmpSat1
  Scope{,1..10} (11 alike) : Scope
  Sensor Gain Q0 : Gain  Gain=Sens0
  Sensor Gain Q1 : Gain  Gain=Sens1
  Sensor Gain Q2 : Gain  Gain=Sens0
  Sensor Gain Q3 : Gain  Gain=Sens1
  Sensor Limit Q0 : Saturate  UpperLimit=SensSat0  LowerLimit=-SensSat0
  Sensor Limit Q1 : Saturate  UpperLimit=SensSat1  LowerLimit=-SensSat1
  Sensor Limit Q2 : Saturate  UpperLimit=SensSat0  LowerLimit=-SensSat0
  Sensor Limit Q3 : Saturate  UpperLimit=SensSat1  LowerLimit=-SensSat1
  Static Friction Q0 : Subsystem
  Static Friction Q1 : Subsystem
  Static Friction Q2 : Subsystem
  Step : Step  Time=0.1  SampleTime=0
  Step1 : Step  Time=0.1  SampleTime=0
  Step2 : Step  SampleTime=0
  Step3 : Step  SampleTime=0
  Sum{,1..4,6,8..11} (10 alike) : Sum  Inputs=|+-
  Sum12 : Sum  Inputs=-+|
  Sum5 : Sum  Inputs=-+|
  Sum7 : Sum  Inputs=-+|
  Torque Const Q0 : Gain  Gain=TConst0
  Torque Const Q1 : Gain  Gain=TConst1
  Torque Const Q2 : Gain  Gain=TConst0
  Torque Const Q3 : Gain  Gain=TConst1
  Torque Const Q4 : Gain  Gain=TConst0
  Torque Const Q5 : Gain  Gain=TConst1
  QaL : Outport
  MotCurr : Outport  Port=2
  wires:
  QdL/1 -> Demux/1
  Mux/1 -> QaL/1
  Controller Q8/1 -> Amplifier Q1/1
  Sum/1 -> Elec Dyn Q1/1
  Sum3/1 -> Controller Q8/1
  Elec Dyn Q1/1 -> Mux1/2, Torque Const Q1/1
  Amplifier Q1/1 -> Saturation Q1/1
  Saturation Q1/1 -> Sum/1
  Back EMF Q1/1 -> Sum/2
  Sensor Gain Q1/1 -> Sensor Limit Q1/1
  Controller Q3/1 -> Amplifier Q0/1
  Sum2/1 -> Controller Q3/1
  Elec Dyn Q0/1 -> Scope/1, Torque Const Q0/1, Mux1/1
  Amplifier Q0/1 -> Scope5/1, Saturation Q0/1
  Saturation Q0/1 -> Sum1/1
  Back EMF Q0/1 -> Scope4/1, Sum1/2
  Sensor Gain Q0/1 -> Sensor Limit Q0/1
  Sum5/1 -> Mech Dyn Q0/1
  Jnt Limit Q1/1 -> Scope6/1, Mux/2, Sensor Gain Q1/1
  Demux/1 -> Sum2/1
  Demux/3 -> Mux/3
  Demux/2 -> Sum3/1
  FB Gain Q0/1 -> Sum2/2
  FB Gain Q1/1 -> Sum3/2
  Static Friction Q0/1(Fout) -> Sum5/1
  Torque Const Q1/1 -> Mech Dyn Q1/1
  Mux1/1 -> MotCurr/1
  Sensor Limit Q1/1 -> FB Gain Q1/1  "(V)"
  Sensor Limit Q0/1 -> FB Gain Q0/1  "(V)"
  Mech Dyn Q0/1 -> Static Friction Q0/2(w), Scope3/1, Integrator Q0/1, Back EMF Q0/1  "rad"
  Integrator Q0/1 -> Scope1/1, Sensor Gain Q0/1, Mux/1
  Integrator Q1/1 -> Scope7/1, Jnt Limit Q1/1
  Torque Const Q0/1 -> Static Friction Q0/1(Fin), Sum5/2
  Mech Dyn Q1/1 -> Integrator Q1/1, Back EMF Q1/1
  Sum1/1 -> Elec Dyn Q0/1
  Static Friction Q1/1(Fout) -> Sum7/1
  Sensor Gain Q2/1 -> Sensor Limit Q2/1
  FB Gain Q2/1 -> Sum6/2
  Saturation Q2/1 -> Sum4/1
  Step/1 -> Sum6/1
  Integrator Q2/1 -> Scope2/1, Sensor Gain Q2/1
  Mech Dyn Q2/1 -> Static Friction Q1/2(w), Integrator Q2/1, Back EMF Q2/1  "rad"
  Sum7/1 -> Mech Dyn Q2/1
  Sum4/1 -> Elec Dyn Q1/1
  Sensor Limit Q2/1 -> FB Gain Q2/1  "(V)"
  Amplifier Q2/1 -> Saturation Q2/1
  Elec Dyn Q1/1 -> Torque Const Q2/1
  Controller Q2/1 -> Amplifier Q2/1
  Back EMF Q2/1 -> Sum4/2
  Sum6/1 -> Controller Q2/1
  Torque Const Q2/1 -> Static Friction Q1/1(Fin), Sum7/2
  Step1/1 -> Sum9/1
  Sensor Gain Q3/1 -> Sensor Limit Q3/1
  Jnt Limit Q2/1 -> Scope8/1, Sensor Gain Q3/1
  Mech Dyn Q3/1 -> Integrator Q3/1, Back EMF Q3/1
  Integrator Q3/1 -> Jnt Limit Q2/1
  Elec Dyn Q2/1 -> Torque Const Q3/1
  Torque Const Q3/1 -> Mech Dyn Q3/1
  Saturation Q3/1 -> Sum8/1
  Sensor Limit Q3/1 -> FB Gain Q3/1  "(V)"
  Sum8/1 -> Elec Dyn Q2/1
  Controller Q5/1 -> Amplifier Q3/1
  Back EMF Q3/1 -> Sum8/2
  Sum9/1 -> Controller Q5/1
  Amplifier Q3/1 -> Saturation Q3/1
  FB Gain Q3/1 -> Sum9/2
  Static Friction Q2/1(Fout) -> Sum12/1
  Saturation Q4/1 -> Sum10/1
  Torque Const Q4/1 -> Static Friction Q2/1(Fin), Sum12/2
  Step2/1 -> Controller Q6/1
  Back EMF Q4/1 -> Sum10/2
  Elec Dyn Q2/1 -> Torque Const Q4/1
  Controller Q6/1 -> Amplifier Q4/1
  Sum10/1 -> Elec Dyn Q2/1
  Amplifier Q4/1 -> Saturation Q4/1
  Integrator Q4/1 -> Scope9/1
  Mech Dyn Q4/1 -> Static Friction Q2/2(w), Integrator Q4/1, Back EMF Q4/1  "rad"
  Sum12/1 -> Mech Dyn Q4/1
  Elec Dyn Q3/1 -> Torque Const Q5/1
  Integrator Q5/1 -> Jnt Limit Q3/1
  Mech Dyn Q5/1 -> Integrator Q5/1, Back EMF Q5/1
  Jnt Limit Q3/1 -> Scope10/1
  Amplifier Q5/1 -> Saturation Q5/1
  Controller Q7/1 -> Amplifier Q5/1
  Step3/1 -> Controller Q7/1
  Torque Const Q5/1 -> Mech Dyn Q5/1
  Back EMF Q5/1 -> Sum11/2
  Sum11/1 -> Elec Dyn Q3/1
  Saturation Q5/1 -> Sum11/1

== system printer/Lamp ==

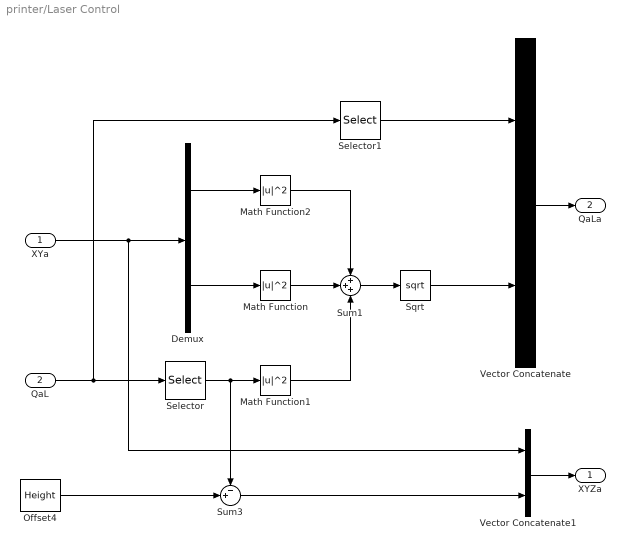
== system printer/Laser Control ==
  XYa : Inport
  QaL : Inport  Port=2
  Demux : Demux  Outputs=2
  Math Function : Math  Operator=magnitude^2  SaturateOnIntegerOverflow=on
  Math Function1 : Math  Operator=magnitude^2  SaturateOnIntegerOverflow=on
  Math Function2 : Math  Operator=magnitude^2  SaturateOnIntegerOverflow=on
  Offset4 : Constant  Value=Height
  Selector : Selector  InputPortWidth=3  IndexOptions=Index vector (dialog)  Indices=3  OutputSizes=1
  Selector1 : Selector  InputPortWidth=3  IndexOptions=Index vector (dialog)  Indices=[1 2]  OutputSizes=1
  Sqrt : Sqrt  SaturateOnIntegerOverflow=on
  Sum1 : Sum  Inputs=+++
  Sum3 : Sum  Inputs=-+|
  Vector Concatenate : Concatenate
  Vector Concatenate1 : Concatenate
  XYZa : Outport
  QaLa : Outport  Port=2
  wires:
  Demux/2 -> Math Function/1
  Demux/1 -> Math Function2/1
  Sqrt/1 -> Vector Concatenate/2
  Math Function2/1 -> Sum1/1
  Math Function/1 -> Sum1/2
  Math Function1/1 -> Sum1/3
  Sum1/1 -> Sqrt/1
  QaL/1 -> Selector1/1, Selector/1
  XYa/1 -> Vector Concatenate1/1, Demux/1
  Selector/1 -> Math Function1/1, Sum3/1
  Selector1/1 -> Vector Concatenate/1
  Vector Concatenate/1 -> QaLa/1
  Vector Concatenate1/1 -> XYZa/1
  Sum3/1 -> Vector Concatenate1/2
  Offset4/1 -> Sum3/2

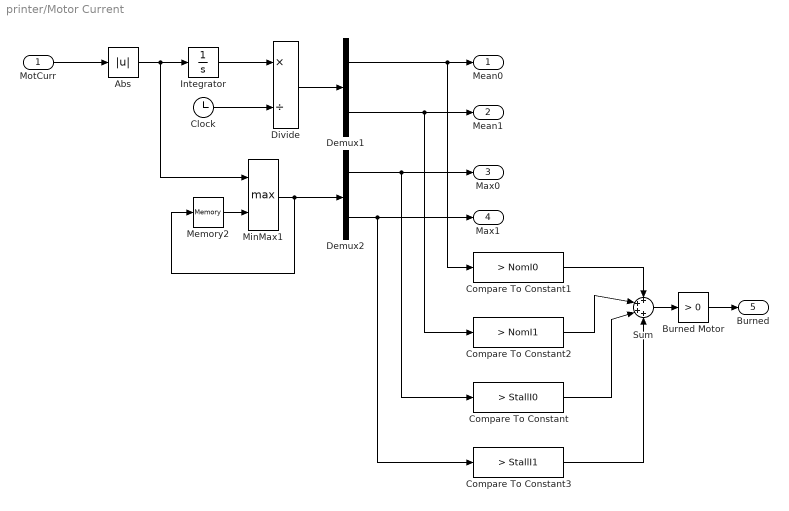
== system printer/Motor Current ==
  MotCurr : Inport
  Abs : Abs
  Burned Motor : simulink/Logic and Bit Operations/Compare To Zero  relop=>  OutDataTypeStr=boolean
  Clock : Clock
  Compare To Constant : simulink/Logic and Bit Operations/Compare To Constant  relop=>  const=StallI0  OutDataTypeStr=boolean
  Compare To Constant1 : simulink/Logic and Bit Operations/Compare To Constant  relop=>  const=NomI0  OutDataTypeStr=boolean
  Compare To Constant2 : simulink/Logic and Bit Operations/Compare To Constant  relop=>  const=NomI1  OutDataTypeStr=boolean
  Compare To Constant3 : simulink/Logic and Bit Operations/Compare To Constant  relop=>  const=StallI1  OutDataTypeStr=boolean
  Demux1 : Demux  Outputs=2
  Demux2 : Demux  Outputs=2
  Divide : Product  Inputs=*/
  Integrator : Integrator
  Memory2 : Memory
  MinMax1 : MinMax  Function=max  Inputs=2
  Sum : Sum  Inputs=++++
  Mean0 : Outport
  Mean1 : Outport  Port=2
  Max0 : Outport  Port=3
  Max1 : Outport  Port=4
  Burned : Outport  Port=5
  wires:
  Demux1/1 -> Compare To Constant1/1, Mean0/1
  MotCurr/1 -> Abs/1
  Integrator/1 -> Divide/1
  Clock/1 -> Divide/2
  Divide/1 -> Demux1/1
  Abs/1 -> MinMax1/1, Integrator/1
  Demux2/1 -> Compare To Constant/1, Max0/1
  Demux1/2 -> Compare To Constant2/1, Mean1/1
  Demux2/2 -> Compare To Constant3/1, Max1/1
  Compare To Constant1/1 -> Sum/1
  Compare To Constant3/1 -> Sum/4
  Compare To Constant/1 -> Sum/3
  Compare To Constant2/1 -> Sum/2
  Memory2/1 -> MinMax1/2
  MinMax1/1 -> Demux2/1, Memory2/1
  Burned Motor/1 -> Burned/1
  Sum/1 -> Burned Motor/1

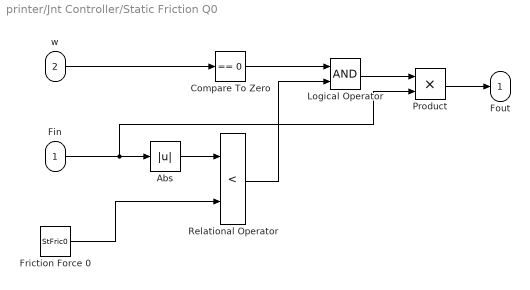
== system printer/Jnt Controller/Static Friction Q0 ==
  Fin : Inport
  w : Inport  Port=2
  Abs : Abs
  Compare To Zero : simulink/Logic and Bit Operations/Compare To Zero  relop===  OutDataTypeStr=boolean
  Friction Force 0 : Constant  Value=StFric0
  Logical Operator : Logic  AllPortsSameDT=off  OutDataTypeStr=boolean
  Product : Product
  Relational Operator : RelationalOperator  Operator=<  OutDataTypeStr=boolean  RndMeth=Simplest
  Fout : Outport
  wires:
  Friction Force 0/1 -> Relational Operator/2
  Product/1 -> Fout/1
  Compare To Zero/1 -> Logical Operator/1
  Relational Operator/1 -> Logical Operator/2
  Logical Operator/1 -> Product/1
  Fin/1 -> Product/2, Abs/1
  w/1 -> Compare To Zero/1
  Abs/1 -> Relational Operator/1

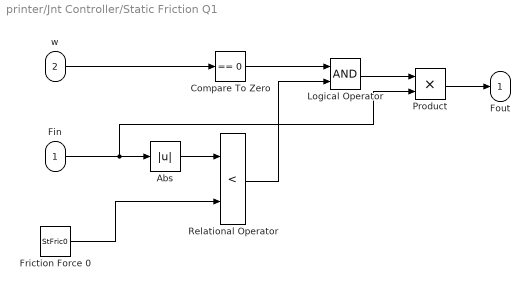
== system printer/Jnt Controller/Static Friction Q1 ==
  Fin : Inport
  w : Inport  Port=2
  Abs : Abs
  Compare To Zero : simulink/Logic and Bit Operations/Compare To Zero  relop===  OutDataTypeStr=boolean
  Friction Force 0 : Constant  Value=StFric0
  Logical Operator : Logic  AllPortsSameDT=off  OutDataTypeStr=boolean
  Product : Product
  Relational Operator : RelationalOperator  Operator=<  OutDataTypeStr=boolean  RndMeth=Simplest
  Fout : Outport
  wires:
  Friction Force 0/1 -> Relational Operator/2
  Product/1 -> Fout/1
  Compare To Zero/1 -> Logical Operator/1
  Relational Operator/1 -> Logical Operator/2
  Logical Operator/1 -> Product/1
  Fin/1 -> Product/2, Abs/1
  w/1 -> Compare To Zero/1
  Abs/1 -> Relational Operator/1

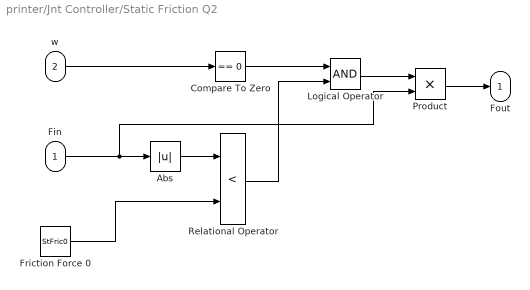
== system printer/Jnt Controller/Static Friction Q2 ==
  Fin : Inport
  w : Inport  Port=2
  Abs : Abs
  Compare To Zero : simulink/Logic and Bit Operations/Compare To Zero  relop===  OutDataTypeStr=boolean
  Friction Force 0 : Constant  Value=StFric0
  Logical Operator : Logic  AllPortsSameDT=off  OutDataTypeStr=boolean
  Product : Product
  Relational Operator : RelationalOperator  Operator=<  OutDataTypeStr=boolean  RndMeth=Simplest
  Fout : Outport
  wires:
  Friction Force 0/1 -> Relational Operator/2
  Product/1 -> Fout/1
  Compare To Zero/1 -> Logical Operator/1
  Relational Operator/1 -> Logical Operator/2
  Logical Operator/1 -> Product/1
  Fin/1 -> Product/2, Abs/1
  w/1 -> Compare To Zero/1
  Abs/1 -> Relational Operator/1
